simulink model "pylab_mini_generator"  (R2020a)
settings: Solver=VariableStepAuto  StartTime=0.0  StopTime=10.0  RelTol=1e-3
model workspace (MAT data in the model file):
  amplitude = Simulink.Parameter
  amplitude.Value = 1
  amplitude.DataType = 'auto'
  amplitude.Dimensions = [1 1]
  bias = Simulink.Parameter
  bias.Value = 0
  bias.DataType = 'auto'
  bias.Dimensions = [1 1]
  constant_value = Simulink.Parameter
  constant_value.Value = 123
  constant_value.DataType = 'auto'
  constant_value.Dimensions = [1 1]
  final_value = Simulink.Parameter
  final_value.Value = 1
  final_value.DataType = 'auto'
  final_value.Dimensions = [1 1]
  frequency = Simulink.Parameter
  frequency.Value = 1
  frequency.DataType = 'auto'
  frequency.Dimensions = [1 1]
  initial_output = Simulink.Parameter
  initial_output.Value = 0
  initial_output.DataType = 'auto'
  initial_output.Dimensions = [1 1]
  initial_value = Simulink.Parameter
  initial_value.Value = 0
  initial_value.DataType = 'auto'
  initial_value.Dimensions = [1 1]
  phase = Simulink.Parameter
  phase.Value = 0
  phase.DataType = 'auto'
  phase.Dimensions = [1 1]
  selection = Simulink.Parameter
  selection.Value = 3
  selection.DataType = 'auto'
  selection.Dimensions = [1 1]
  slope = Simulink.Parameter
  slope.Value = 1
  slope.DataType = 'auto'
  slope.Dimensions = [1 1]
  start_time = Simulink.Parameter
  start_time.Value = 0
  start_time.DataType = 'auto'
  start_time.Dimensions = [1 1]
  step_time = Simulink.Parameter
  step_time.Value = 0
  step_time.DataType = 'auto'
  step_time.Dimensions = [1 1]
libraries: simulink x1
settings Model: ParameterArgumentNames=constant_value,amplitude,bias,frequency,phase,slope,start_time,initial_output,step_time,initial_value,final_value,selection  Creator=malte  LastModifiedBy=malte

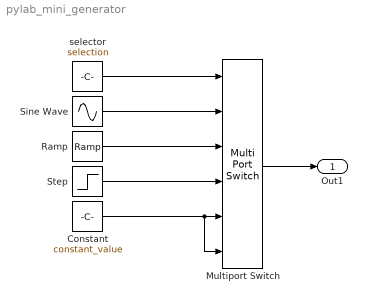
== system pylab_mini_generator ==
  Constant : Constant  Value=constant_value
  Multiport Switch : MultiPortSwitch  DataPortOrder=Zero-based contiguous  Inputs=4  DataPortForDefault=Additional data port  DiagnosticForDefault=None  zeroidx=on
  Ramp : simulink/Sources/Ramp  slope=slope  start=start_time  InitialOutput=initial_output
  Sine Wave : Sin  Amplitude=amplitude  Bias=bias  Frequency=frequency  Phase=phase  SampleTime=0
  Step : Step  Time=step_time  Before=initial_value  After=final_value  SampleTime=0
  selector : Constant  Value=selection
  Out1 : Outport
  wires:
  Sine Wave/1 -> Multiport Switch/2
  Ramp/1 -> Multiport Switch/3
  Step/1 -> Multiport Switch/4
  Multiport Switch/1 -> Out1/1
  selector/1 -> Multiport Switch/1
  Constant/1 -> Multiport Switch/6, Multiport Switch/5
